simulink model "Sim2"  (R2022a)
settings: Solver=FixedStepAuto  StartTime=0.0  StopTime=100  FixedStep=0.01  RelTol=1e-3
values from neighbouring files (symbols this model uses):
  K_dx = 0.04    [sim_init.m]
  K_x = 0.02    [sim_init.m]
  Kd = 0.8    [sim_init.m]
  Kp = 3.5    [sim_init.m]
  q0 = [1,0,-0.3,0]'    [sim_init.m]
  x_des = 0    [sim_init.m]
settings Model: Creator=ariannagasparri  LastModifiedBy=Marco
settings SolverCC: AlgebraicLoopSolver=TrustRegion
settings DebuggingCC: AlgebraicLoopMsg=none  UnconnectedInputMsg=warning  UnconnectedOutputMsg=warning  UnconnectedLineMsg=warning  SFMachineParentedDataDiag=warning

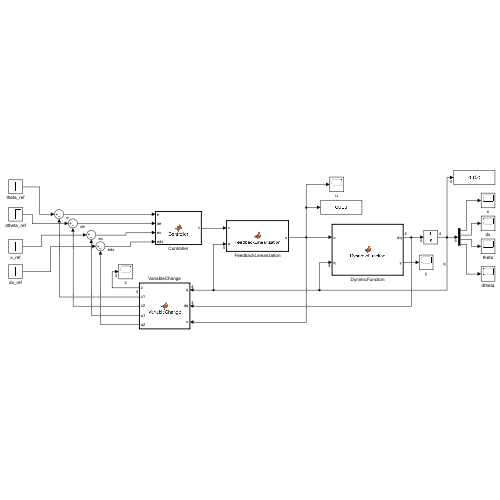
[thumbnail: Simulink's stored preview of the top-level diagram]
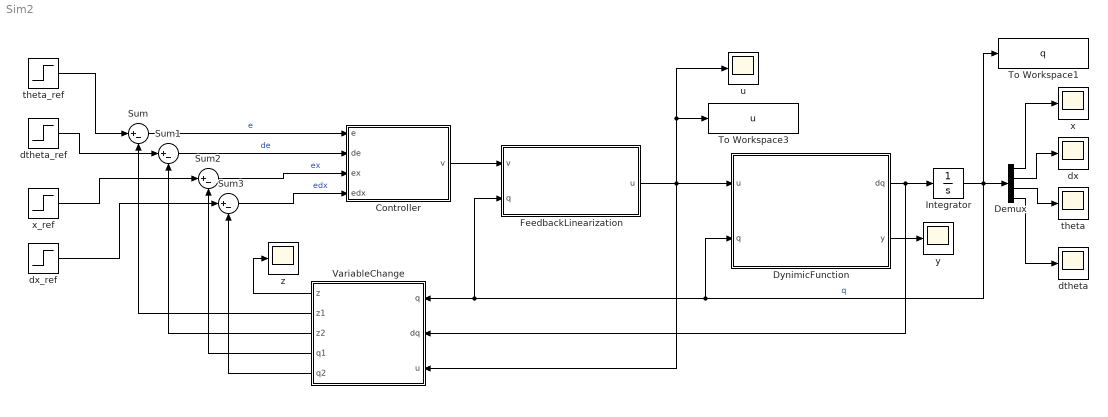
== system Sim2 ==
  Controller : MATLAB Function  TreatAsAtomicUnit=on
  Demux : Demux
  DynimicFunction : MATLAB Function  TreatAsAtomicUnit=on
  FeedbackLinearization : MATLAB Function  TreatAsAtomicUnit=on
  Integrator : Integrator  InitialCondition=q0
  Sum{,1..3} (4 alike) : Sum  Inputs=|+-
  To Workspace1 : ToWorkspace  VariableName=q  SaveFormat=Timeseries  SampleTime=-1
  To Workspace3 : ToWorkspace  VariableName=u  SaveFormat=Timeseries  SampleTime=-1
  VariableChange : MATLAB Function  TreatAsAtomicUnit=on
  dtheta : Scope
  dtheta_ref : Step  Time=0  After=0  SampleTime=0
  dx : Scope
  dx_ref : Step  Time=0  After=0  SampleTime=0
  theta : Scope
  theta_ref : Step  Time=0  After=0  SampleTime=0
  u : Scope
  x : Scope
  x_ref : Step  Time=0  After=x_des  SampleTime=0
  y : Scope
  z : Scope
  wires:
  DynimicFunction/1(dq) -> Integrator/1, VariableChange/2(dq)
  Sum/1 -> Controller/1(e)  "e"
  Controller/1(v) -> FeedbackLinearization/1(v)
  VariableChange/1(z) -> z/1
  Sum1/1 -> Controller/2(de)  "de"
  Demux/3 -> theta/1
  Demux/1 -> x/1
  Demux/2 -> dx/1
  Integrator/1 -> To Workspace1/1, Demux/1, DynimicFunction/2(q), FeedbackLinearization/2(q), VariableChange/1(q)  "q"
  Demux/4 -> dtheta/1
  dtheta_ref/1 -> Sum1/1
  FeedbackLinearization/1(u) -> VariableChange/3(u), DynimicFunction/1(u), To Workspace3/1, u/1
  VariableChange/2(z1) -> Sum/2
  VariableChange/3(z2) -> Sum1/2
  theta_ref/1 -> Sum/1
  Sum3/1 -> Controller/4(edx)  "edx"
  Sum2/1 -> Controller/3(ex)  "ex"
  VariableChange/4(q1) -> Sum2/2
  x_ref/1 -> Sum2/1
  VariableChange/5(q2) -> Sum3/2
  dx_ref/1 -> Sum3/1
  DynimicFunction/2(y) -> y/1

== matlab function Sim2/FeedbackLinearization ==
  data: v input; u output; q input; param parameter
function u = FeedbackLinearization(v, q, param)

    M = param(1);
    m = param(2);
    l = param(3);
    gravity = param(4);
    b = param(5);
    
    u = ((M+m)*gravity*sin(q(3))+b*q(2)*cos(q(3))-m*l*cos(q(3))*sin(q(3))*q(4)^2)/cos(q(3))-l*v*(M+m*sin(q(3))^2)/cos(q(3)) ;

end

== matlab function Sim2/DynimicFunction ==
  data: u input; dq output; q input; y output; param parameter
function [dq, y] = DynamicFunction(u, q, param)

    M = param(1);
    m = param(2);
    l = param(3);
    gravity = param(4);
    b = param(5);
    
    dq = f_fun(M,b,gravity,l,m,q) + g_fun(M,l,m,q)*u;
    
    y = h_fun(q);

end

== matlab function Sim2/VariableChange ==
  data: q input; dq input; z output; u input; z1 output; z2 output; param parameter; q1 output; q2 output
function [z,z1,z2,q1,q2]   = VariableChange(q, dq, u, param)

    z = zeros(4,1);
    dz = zeros(4,1);
    
    M = param(1);
    m = param(2);
    l = param(3);
    gravity = param(4);
    b = param(5);
    
    z(1) = q(3);
    z(2) = q(4);
    z(3) = q(1);
    z(4) = q(2)*cos(q(3)) + l*q(4);
    
    % dz(1) = z(2);
    % dz(2) = dq(1);
    % dz(3) = Lf2h + LgLfh*u; % = v
    % dz(4) = jacobian(z(4),q)*dq;
    
    z1 = z(1);
    z2 = z(2);

    q1 = q(1);
    q2 = q(2);

end

== matlab function Sim2/Controller ==
  data: e input; de input; v output; Kp parameter; Kd parameter; ex input; edx input; K_x parameter; K_dx parameter
function v = Controller(e, de, Kp, Kd, ex, edx, K_x, K_dx)

    % Controllo stabilizzante anche posizione
    v = (Kp * e + Kd * de) + K_x*ex + K_dx*edx;
    
    % Controllo stabilizzante solo angolo
    % v = (Kp * e + Kd * de)

end
